simulink model "Systemidentifikation"  (Simulink 8.7)
settings: Solver=ode4  StartTime=0.0  StopTime=40  FixedStep=0.001  RelTol=1e-3
settings Model: Creator=roth  LastModifiedBy=Oliver
settings DebuggingCC: UnderspecifiedInitializationDetection=Simplified  MergeDetectMultiDrivingBlocksExec=error  SolverPrmCheckMsg=warning
settings ConfigComp: CovSFcnEnable=off

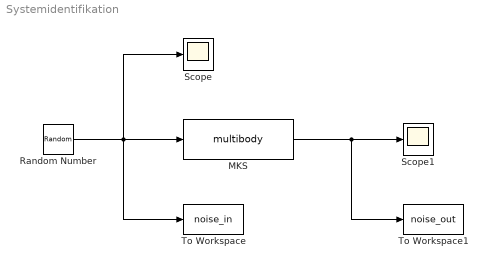
== system Systemidentifikation ==
  MKS : S-Function  FunctionName=multibody  Parameters='Kiethe'  SFunctionDeploymentMode=off  EnableBusSupport=off
  Random Number : RandomNumber  Seed=123456789  SampleTime=0.001
  Scope : Scope
  Scope1 : Scope
  To Workspace : ToWorkspace  VariableName=noise_in  SaveFormat=Timeseries  SampleTime=-1
  To Workspace1 : ToWorkspace  VariableName=noise_out  SaveFormat=Timeseries  SampleTime=-1
  wires:
  MKS/1 -> To Workspace1/1, Scope1/1
  Random Number/1 -> To Workspace/1, Scope/1, MKS/1
